simulink model "Continuous_PID"  (R2022a)
settings: Solver=ode4  StartTime=0.0  StopTime=20  FixedStep=0.001  RelTol=1e-3
values from neighbouring files (symbols this model uses):
  kd = 0    [ContinuousPID.m]
  ki = 0    [ContinuousPID.m]
  kp = 1    [ContinuousPID.m]
libraries: cstblocks x1
settings Model: Creator=David  LastModifiedBy=David

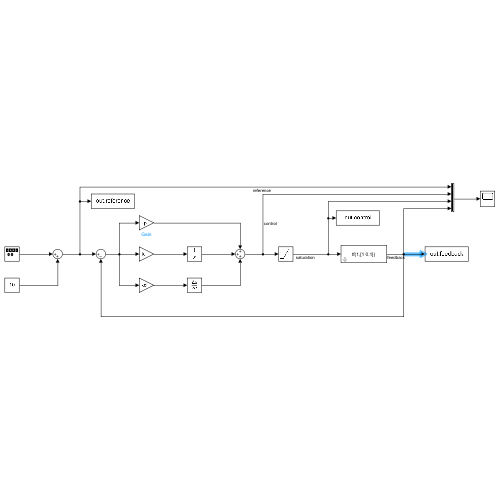
[thumbnail: Simulink's stored preview of the top-level diagram]
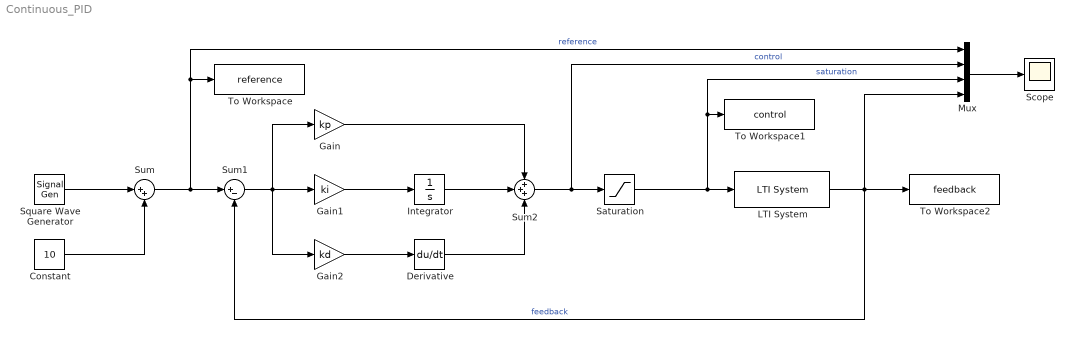
== system Continuous_PID ==
  Constant : Constant  Value=10
  Derivative : Derivative
  Gain : Gain  Gain=kp
  Gain1 : Gain  Gain=ki
  Gain2 : Gain  Gain=kd
  Integrator : Integrator
  LTI System : cstblocks/LTI System  sys=tf(1,[1 0.1])  IC=[]
  Mux : Mux
  Saturation : Saturate  UpperLimit=2^31-1  LowerLimit=-2^31
  Scope : Scope
  Square Wave Generator : SignalGenerator  WaveForm=square  Amplitude=10  Frequency=0.1
  Sum : Sum  Inputs=|++
  Sum1 : Sum  Inputs=|+-
  Sum2 : Sum  Inputs=+++
  To Workspace : ToWorkspace  VariableName=reference  SampleTime=-1
  To Workspace1 : ToWorkspace  VariableName=control  SampleTime=-1
  To Workspace2 : ToWorkspace  VariableName=feedback  SampleTime=-1
  wires:
  Square Wave Generator/1 -> Sum/1
  Constant/1 -> Sum/2
  Sum/1 -> To Workspace/1, Mux/1, Sum1/1  "reference"
  Sum1/1 -> Gain2/1, Gain/1, Gain1/1
  Gain1/1 -> Integrator/1
  Gain2/1 -> Derivative/1
  Sum2/1 -> Mux/2, Saturation/1  "control"
  Mux/1 -> Scope/1
  Saturation/1 -> To Workspace1/1, Mux/3, LTI System/1  "saturation"
  LTI System/1 -> Sum1/2, To Workspace2/1, Mux/4  "feedback"
  Gain/1 -> Sum2/1
  Integrator/1 -> Sum2/2
  Derivative/1 -> Sum2/3
